simulink model "temp_vehicle"  (R2018a)
settings: Solver=ode45  StartTime=0.0  StopTime=inf  FixedStep=0.1  RelTol=1e-3  EnableMultiTasking=on
PreLoadFcn:
  | RTWConfigurationCB('preloadfcn', bdroot);
InitFcn:
  | parameterVehicle
StopFcn:
  | myStopFcnExperiment(xAct,yAct)
values from neighbouring files (symbols this model uses):
  b = 0.56488    [parameterVehicle.m]
  dcArray = [-100 -11 -10 0 10 11 100]    [parameterVehicle.m]
  eTick = 4384    [parameterVehicle.m]
  rl = 1.0013040494*rNominal    (= 0.0617601003327)    [parameterVehicle.m]
  rr = 0.9986959506*rNominal    (= 0.0615992336673)    [parameterVehicle.m]
  thetaIC = 0*(pi/180)    (= 0)    [parameterVehicle.m]
  TsampleEncoder = 1/10    (= 0.1)    [parameterVehicle.m]
  wArray = [-Vmax, -Vmin, 0, 0,   0, Vmin, Vmax]./rNominal    [parameterVehicle.m]
  xIC = 0    [parameterVehicle.m]
  yIC = 0    [parameterVehicle.m]
libraries: robotlib x6, dspsigops x1, simulink x1
CloseFcn:
  | rtwprivate ssgencode ModelCloseRequest track_vehicle6_v2
settings Model: Creator=Dogan  LastModifiedBy=askar
settings DataIOCC: LimitDataPoints=on  SaveFormat=Array  SignalLoggingSaveFormat=ModelDataLogs
settings OptimizationCC: ExpressionDepthLimit=2147483647  InitFltsAndDblsToZero=on  LifeSpan=1
settings DebuggingCC: SaveWithParameterizedLinksMsg=none  UnderspecifiedInitializationDetection=Classic  MergeDetectMultiDrivingBlocksExec=none  SignalResolutionControl=TryResolveAllWithWarning  SolverPrmCheckMsg=warning  MultiTaskDSMMsg=warning  MultiTaskCondExecSysMsg=none  FcnCallInpInsideContextMsg=warning  StateNameClashWarn=warning  SFUnexpectedBacktrackingDiag=warning  SFNoUnconditionalDefaultTransitionDiag=warning  SFExecutionAtInitializationDiag=none
settings HardwareCC: ProdBitPerPointer=32  ProdBitPerSizeT=32  ProdBitPerPtrDiffT=32  ProdLargestAtomicInteger=Long  ProdLargestAtomicFloat=Double  ProdEndianess=BigEndian  ProdWordSize=32  ProdHWDeviceType=Motorola PowerPC  TargetHWDeviceType=32-bit Generic
settings ModelReferenceCC: PropagateSignalLabelsOutOfModel=off
settings SFSimCC: SimParseCustomCode=off  MATLABDynamicMemAlloc=off
settings RTWCC: SystemTargetFile=mpc555rt.tlc  TemplateMakefile=mpc555rt.tmf  Description=Target for Freescale MPC5xx (real-time)
settings CodeAppCC: GenerateComments=off  IgnoreCustomStorageClasses=off  CustomSymbolStrType=$N$R$M  SimulinkBlockComments=off  InternalIdentifier=Classic
settings STFCustomTargetCC: TargetLibSuffix=.a  IncludeMdlTerminateFcn=off  CombineOutputUpdateFcns=on  ERTCustomFileBanners=on  SupportNonFinite=off  SupportContinuousTime=off  SupportNonInlinedSFcns=off  RemoveResetFunc=on  MATLABClassNameForMDSCustomization=Simulink.SoftwareTarget.ERTCustomization  CPPClassGenCompliant=on  GRTInterface=off  SystemTargetFile=mpc555rt.tlc
settings ERTTargetCC: MultiwordLength=2048  ParMdlRefBuildCompliant=off  CompOptLevelCompliant=off  ConcurrentExecutionCompliant=off  IncludeMdlTerminateFcn=off  SupportNonFinite=off  ModelStepFunctionPrototypeControlCompliant=off  UseToolchainInfoCompliant=off  ExtModeMexFile=MPC5xxExternalModeOpen  ExtModeIntrfLevel=Level2 - Open  ERTCustomFileTemplate=example_file_process.tlc  ConvertIfToSwitch=off  SuppressUnreachableDefaultCases=off
settings ConfigComp: CovMetricSettings=dw  CovHtmlReporting=on  CovSaveCumulativeToWorkspaceVar=on  CovSaveSingleToWorkspaceVar=on  CovExternalEMLEnable=off

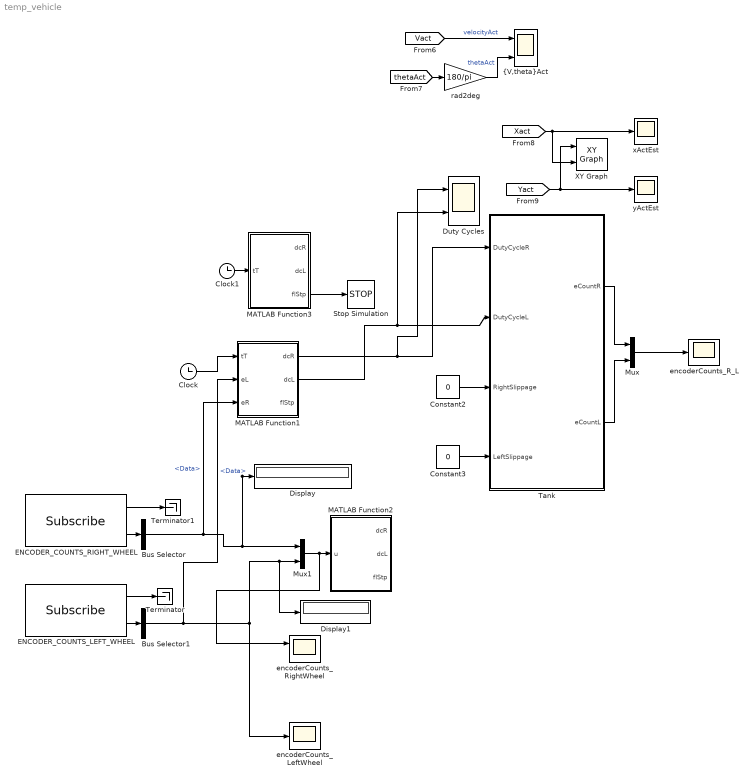
== system temp_vehicle ==
  Bus Selector : BusSelector  OutputSignals=Data
  Bus Selector1 : BusSelector  OutputSignals=Data
  Clock : Clock
  Clock1 : Clock
  Constant2 : Constant  Value=0
  Constant3 : Constant  Value=0
  Display : Display
  Display1 : Display
  Duty Cycles : Scope  NumInputPorts=2
  ENCODER_COUNTS_LEFT_WHEEL : robotlib/Subscribe  SourceLibraryInfo=This block requires Robotics System Toolbox  topicSource=Select from ROS network  topic=/enco_L  messageType=std_msgs/Int16  sampleTime=-1  messageQueueLength=1
      settings: SourceProductBaseCode=RO
  ENCODER_COUNTS_RIGHT_WHEEL : robotlib/Subscribe  SourceLibraryInfo=This block requires Robotics System Toolbox  topicSource=Select from ROS network  topic=/enco_R  messageType=std_msgs/Int16  sampleTime=-1  messageQueueLength=1
      settings: SourceProductBaseCode=RO
  MATLAB Function1 : MATLAB Function  TreatAsAtomicUnit=on
  MATLAB Function2 : MATLAB Function  TreatAsAtomicUnit=on
  MATLAB Function3 : MATLAB Function  TreatAsAtomicUnit=on
  Mux : Mux  Inputs=2
  Mux1 : Mux  Inputs=2
  Stop Simulation : Stop
  Tank : Subsystem
  Terminator : Terminator
  Terminator1 : Terminator
  XY Graph : simulink/Sinks/XY Graph  xmin=-7  xmax=20  ymin=-7  ymax=18  st=-1
  encoderCounts_LeftWheel : Scope
  encoderCounts_R_L : Scope
  encoderCounts_RightWheel : Scope  NumInputPorts=2
  rad2deg : Gain  Gain=180/pi
  xActEst : Scope
  yActEst : Scope
  "{V,theta}Act" : Scope  NumInputPorts=2
  wires:
  Constant2/1 -> Tank/3(RightSlippage)
  Constant3/1 -> Tank/4(LeftSlippage)
  Tank/2(eCountL) -> Mux/2
  Tank/1(eCountR) -> Mux/1
  rad2deg/1 -> "{V,theta}Act"/2  "thetaAct"
  [Vact] -> "{V,theta}Act"/1  "velocityAct"
  [thetaAct] -> rad2deg/1
  [Xact] -> xActEst/1, XY Graph/2
  [Yact] -> XY Graph/1, yActEst/1
  MATLAB Function3/3(flStp) -> Stop Simulation/1
  Clock/1 -> MATLAB Function1/1(tT)
  Clock1/1 -> MATLAB Function3/1(tT)
  Mux/1 -> encoderCounts_R_L/1
  ENCODER_COUNTS_LEFT_WHEEL/2 -> Bus Selector1/1
  ENCODER_COUNTS_RIGHT_WHEEL/1 -> Terminator1/1
  Bus Selector1/1 -> MATLAB Function1/2(eL), encoderCounts_LeftWheel/1, Display1/1, Mux1/2  "<Data>"
  ENCODER_COUNTS_LEFT_WHEEL/1 -> Terminator/1
  Bus Selector/1 -> MATLAB Function1/3(eR), Mux1/1, Display/1  "<Data>"
  ENCODER_COUNTS_RIGHT_WHEEL/2 -> Bus Selector/1
  Mux1/1 -> encoderCounts_RightWheel/1, MATLAB Function2/1(u)
  MATLAB Function1/1(dcR) -> Duty Cycles/1, Tank/1(DutyCycleR)
  MATLAB Function1/2(dcL) -> Duty Cycles/2, Tank/2(DutyCycleL)

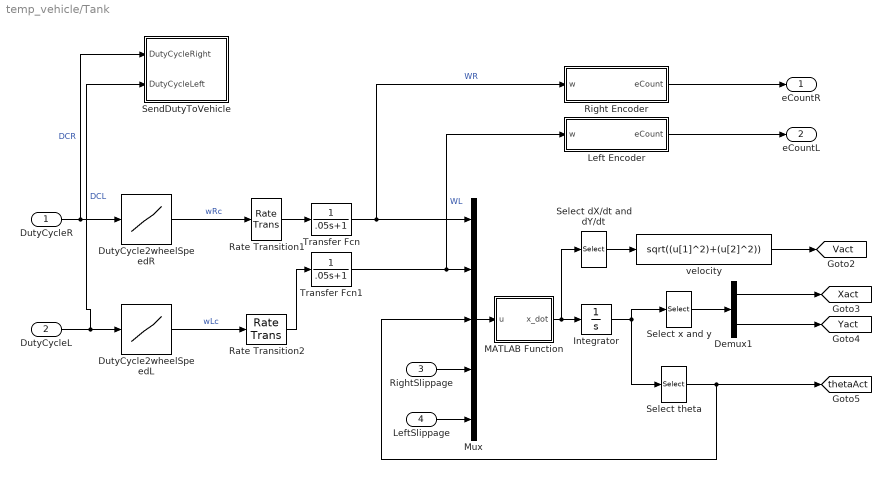
== system temp_vehicle/Tank ==
  DutyCycleR : Inport
  DutyCycleL : Inport  Port=2
  RightSlippage : Inport  Port=3
  LeftSlippage : Inport  Port=4
  Demux1 : Demux  Outputs=2
  DutyCycle2wheelSpeedL : Lookup  InputValues=dcArray  Table=wArray  LookUpMeth=Interpolation-Use End Values
  DutyCycle2wheelSpeedR : Lookup  InputValues=dcArray  Table=wArray  LookUpMeth=Interpolation-Use End Values
  Integrator : Integrator  InitialCondition=[xIC; yIC ; thetaIC]
  Left Encoder : Subsystem
  MATLAB Function : MATLAB Function  TreatAsAtomicUnit=on
  Mux : Mux  Inputs=5
  Rate Transition1 : RateTransition
  Rate Transition2 : RateTransition
  Right Encoder : Subsystem
  Select dX/dt and dY/dt : Selector  InputPortWidth=3  IndexOptions=Index vector (dialog)  Indices=[1 2]  OutputSizes=1
  Select theta : Selector  InputPortWidth=3  IndexOptions=Index vector (dialog)  Indices=3  OutputSizes=1
  Select x and y : Selector  InputPortWidth=3  IndexOptions=Index vector (dialog)  Indices=[1 2]  OutputSizes=1
  SendDutyToVehicle : Subsystem
  Transfer Fcn : TransferFcn  Denominator=[.05 1]
  Transfer Fcn1 : TransferFcn  Denominator=[.05 1]
  velocity : Fcn  Expr=sqrt((u[1]^2)+(u[2]^2))
  eCountR : Outport
  eCountL : Outport  Port=2
  tag scope: Vact=global, Xact=global, Yact=global, thetaAct=global
  wires:
  Integrator/1 -> Select theta/1, Select x and y/1
  Mux/1 -> MATLAB Function/1(u)
  RightSlippage/1 -> Mux/4
  LeftSlippage/1 -> Mux/5
  Transfer Fcn/1 -> Mux/1, Right Encoder/1(w)  "WR"
  Transfer Fcn1/1 -> Mux/2, Left Encoder/1(w)  "WL"
  Select theta/1 -> Mux/3, [thetaAct]
  MATLAB Function/1(x_dot) -> Select dX/dt and dY/dt/1, Integrator/1
  Select dX/dt and dY/dt/1 -> velocity/1
  velocity/1 -> [Vact]
  Select x and y/1 -> Demux1/1
  Demux1/1 -> [Xact]
  Demux1/2 -> [Yact]
  Rate Transition1/1 -> Transfer Fcn/1
  Rate Transition2/1 -> Transfer Fcn1/1
  Left Encoder/1(eCount) -> eCountL/1
  Right Encoder/1(eCount) -> eCountR/1
  DutyCycle2wheelSpeedR/1 -> Rate Transition1/1  "wRc"
  DutyCycle2wheelSpeedL/1 -> Rate Transition2/1  "wLc"
  DutyCycleR/1 -> SendDutyToVehicle/1(DutyCycleRight), DutyCycle2wheelSpeedR/1  "DCR"
  DutyCycleL/1 -> SendDutyToVehicle/2(DutyCycleLeft), DutyCycle2wheelSpeedL/1  "DCL"

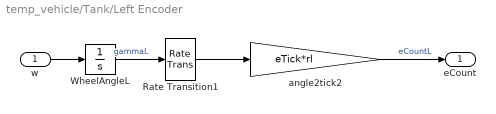
== system temp_vehicle/Tank/Left Encoder ==
  w : Inport
  Rate Transition1 : RateTransition
  WheelAngleL : Integrator
  angle2tick2 : Gain  Gain=eTick*rl  OutDataTypeStr=int16  SampleTime=TsampleEncoder
  eCount : Outport
  wires:
  WheelAngleL/1 -> Rate Transition1/1  "gammaL"
  w/1 -> WheelAngleL/1
  angle2tick2/1 -> eCount/1  "eCountL"
  Rate Transition1/1 -> angle2tick2/1

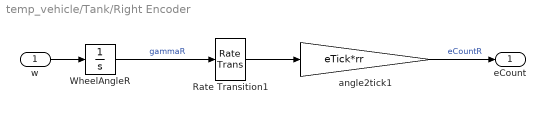
== system temp_vehicle/Tank/Right Encoder ==
  w : Inport
  Rate Transition1 : RateTransition
  WheelAngleR : Integrator
  angle2tick1 : Gain  Gain=eTick*rr  OutDataTypeStr=int16  SampleTime=TsampleEncoder
  eCount : Outport
  wires:
  WheelAngleR/1 -> Rate Transition1/1  "gammaR"
  w/1 -> WheelAngleR/1
  angle2tick1/1 -> eCount/1  "eCountR"
  Rate Transition1/1 -> angle2tick1/1

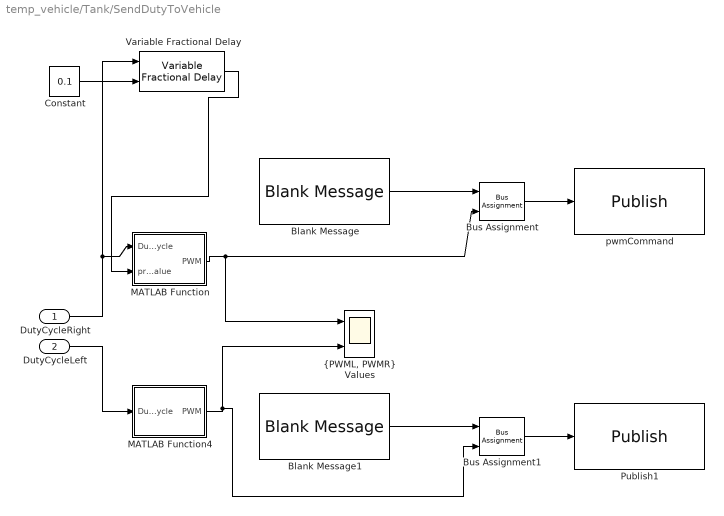
== system temp_vehicle/Tank/SendDutyToVehicle ==
  DutyCycleRight : Inport
  DutyCycleLeft : Inport  Port=2
  Blank Message : robotlib/Blank Message  SourceLibraryInfo=This block requires Robotics System Toolbox  messageType=std_msgs/Int16  SampleTime=inf
      settings: SourceProductBaseCode=RO
  Blank Message1 : robotlib/Blank Message  SourceLibraryInfo=This block requires Robotics System Toolbox  messageType=std_msgs/Int16  SampleTime=inf
      settings: SourceProductBaseCode=RO
  Bus Assignment : BusAssignment  AssignedSignals=Data
  Bus Assignment1 : BusAssignment  AssignedSignals=Data
  Constant : Constant  Value=0.1
  MATLAB Function : MATLAB Function  TreatAsAtomicUnit=on
  MATLAB Function4 : MATLAB Function  TreatAsAtomicUnit=on
  Publish1 : robotlib/Publish  SourceLibraryInfo=This block requires Robotics System Toolbox  topicSource=Select from ROS network  topic=/pwm_cmd_l  messageType=std_msgs/Int16  messageQueueLength=1
      settings: SourceProductBaseCode=RO
  Variable Fractional Delay : dspsigops/Variable Fractional Delay  mode=OBSOLETE  modeActive=Linear  dmax=100  InputProcessing=Columns as channels (frame based)  L=4  FarrowL=4  R=10  alpha=1  ic=0  fallbackFIR=Clip to the minimum value necessary for centered kernel  fallbackFarrow=Clip to the minimum value necessary for centered kernel  noDFT=off  roundingMode=Zero  overflowMode=off
      settings: SourceProductName=DSP System Toolbox  SourceProductBaseCode=DS
  pwmCommand : robotlib/Publish  SourceLibraryInfo=This block requires Robotics System Toolbox  topicSource=Select from ROS network  topic=/pwm_cmd_r  messageType=std_msgs/Int16  messageQueueLength=1
      settings: SourceProductBaseCode=RO
  "{PWML, PWMR} Values" : Scope  NumInputPorts=2
  wires:
  DutyCycleLeft/1 -> MATLAB Function4/1(DutyCycle)
  DutyCycleRight/1 -> Variable Fractional Delay/1, MATLAB Function/1(DutyCycle)
  Blank Message/1 -> Bus Assignment/1
  MATLAB Function4/1(PWM) -> Bus Assignment1/2, "{PWML, PWMR} Values"/2
  MATLAB Function/1(PWM) -> Bus Assignment/2, "{PWML, PWMR} Values"/1
  Bus Assignment/1 -> pwmCommand/1
  Bus Assignment1/1 -> Publish1/1
  Blank Message1/1 -> Bus Assignment1/1
  Variable Fractional Delay/1 -> MATLAB Function/2(previousValue)
  Constant/1 -> Variable Fractional Delay/2

== matlab function temp_vehicle/Tank/MATLAB Function ==
  data: u input; x_dot output; b parameter; rr parameter; rl parameter
function x_dot = fcn(u,b,rr,rl)
%#codegen

wr = u(1);
wl = u(2);
theta = u(3);
sr = u(4);
sl = u(5);
x_dot = [((1-sl)*rl*wl + (1-sr)*rr*wr)*cos(theta)/2;
         ((1-sl)*rl*wl + (1-sr)*rr*wr)*sin(theta)/2;
         ((1-sl)*rl*wl - (1-sr)*rr*wr)/b];

== matlab function temp_vehicle/MATLAB Function3 ==
  data: tT input; dcR output; dcL output; flStp output
function [dcR,dcL,flStp] = lookUptableEst(tT)
%#codegen

dcR = 0;
dcL = 0;
flStp = 1;

if tT < 30
    dcR = 30;
    dcL = 30;    
    flStp = 0;    
end

== matlab function temp_vehicle/MATLAB Function1 ==
  data: tT input; dcR output; dcL output; flStp output; eL input; eR input
function [dcR,dcL,flStp] = bTest(tT, eL, eR)
%#codegen

dcR = 30;
dcL = 30;
flStp = 0;

if tT >= 3 && tT < 7
    dcR = 60;
    dcL = 30;
    if tT == 3
        disp(eL)
        disp(eR)
    end
    
elseif tT > 3
    dcR = 0;
    dcL = 0;
    flStp = 1;    
end

== matlab function temp_vehicle/MATLAB Function2 ==
  data: u input; dcR output; dcL output; flStp output
function [dcR,dcL,flStp] = eTickTest(u)
%#codegen

dcR = 0;
dcL = 0;
flStp = 1;
if u(1) < 22212 && u(2) < 22212
    dcR = 30;
    dcL = 30;
else
    dcR = 0;
    dcL = 0;
% 
% if u(2) < 300
%     dcL = 30;
% else
%     dcL = 0;
end

% %%%
% if u(1) > 0
%     dcR = -30;
%     %dcL = -30;
%     flStp = 0;
% elseif u(1) < 0
%     dcR = 30;
% else 
%     dcR = 0;
%     %dcL = 0;
% end
% if u(2) > 0
%     dcL = -30;
% elseif u(2) < 0
%     dcL = 30;
% else
%     %dcR = 0;
%     dcL = 0;
% %%%
end

== matlab function temp_vehicle/Tank/SendDutyToVehicle/MATLAB Function ==
  data: DutyCycle input; PWM output; previousValue input
function PWM = fcn(DutyCycle, previousValue)
    if DutyCycle == 0 && previousValue > 0
        PWM = int16(previousValue - 10);
        disp([DutyCycle previousValue])
    else
        PWM = int16(DutyCycle/100 * 255);
    end

== matlab function temp_vehicle/Tank/SendDutyToVehicle/MATLAB Function4 ==
  data: DutyCycle input; PWM output
function PWM = fcn(DutyCycle)

    PWM = int16(DutyCycle/100 * 255);
